simulink library "lib_drive_cycle2"  (Simulink 5.1)
values from neighbouring files (symbols this model uses):
  logFlag = 1    [advSACompMaskInit.m]    (also in advSACompMaskInitR13.m)
undefined symbols (not defined in the file or in its folder): cyc_avg_time, cyc_cargo_mass, cyc_elevation_init, cyc_filter_bool, cyc_grade, cyc_mph, veh_mass
libraries: lib_drive_cycle x2
settings Model: LastModifiedBy=mokeefe  ProdHWDeviceType=Microprocessor
settings Model: ModifiedComment=|
  | mokeefe -- Thu Apr 18 08:26:19 2002 -- Version 1.14
  | saving the model:
  | o "without the model browser open"
  | o with only top-level screen visible
  | o with "fit to view" enabled
  | o with "status bar" off and "toolbar" off
  | o with "prompt to update model history with each save" on
settings Model: ModifiedHistory=|
  | mokeefe -- Thu Apr 18 08:26:19 2002 -- Version 1.14
  | saving the model:
  | o "without the model browser open"
  | o with only top-level screen visible
  | o with "fit to view" enabled
  | o with "status bar" off and "toolbar" off
  | o with "prompt to update model history with each save" on
  | 
  | mokeefe -- Thu Apr 18 08:26:19 2002 -- Version 1.14
  | saving the model:
  | o "without the model browser open"
  | o with only top-level screen visible
  | o with "fit to view" enabled
  | o with "status bar" off and "toolbar" off
  | o with "prompt to update model history with each save" on
  | 
  | mokeefe -- Thu Apr 18 08:26:08 2002 -- Version 1.13
  | saving the model:
  | o "without the model browser open"
  | o with only top-level screen visible
  | o with "fit to view" enabled
  | o with "status bar" off and "toolbar" off
  | o with "prompt to update model history with each save" on

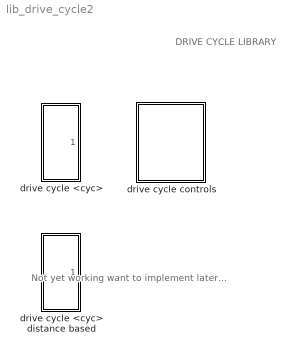
== system lib_drive_cycle2 ==
  note: DRIVE CYCLE LIBRARY
  note: Not yet working
      | want to implement
      | later...
  drive cycle <cyc> : Subsystem  mask(Stand-Alone Drive Cycle Mask){generalName='cyc', logPick=Log, initFileName={}, modCell={}, imgFileName='bdi_cyc.jpg', DEBUG=OFF, veh_mass=veh_mass}
      mask prompts: generalName "General Name of this Component [char]"; logPick "Log Variables to Workspace?"; initFileName "Initialization File(s) [cell array of char]"; modCell "Modification Cell [2 column cell array of param and val]"; imgFileName "Icon image file name [char--evaluated]"; veh_mass "Vehicle Mass (kg)"
      mask init:
      | % initialization via m-file script
      | advSACompMaskInitR13;
      mask StyleString: edit,popup(Don't Log|Log),edit,edit,edit,popup(ON|OFF),edit
      mask Display: image(imread(imgFileName))
  drive cycle <cyc> distance based : Subsystem  mask(Stand-Alone Distance-Based Drive Cycle Mask){generalName='cycd', logPick=Log, initFileName={}, modCell={}, imgFileName='bdi_cyc.jpg', DEBUG=OFF, veh_mass=veh_mass}
      mask prompts: generalName "General Name of this Component [char]"; logPick "Log Variables to Workspace?"; initFileName "Initialization File(s) [cell array of char]"; modCell "Modification Cell [2 column cell array of param and val]"; imgFileName "Icon image file name [char--evaluated]"; veh_mass "Vehicle Mass (kg)"
      mask init:
      | set_param(gcs,'StopTime','inf'); % set stop time to inf
      | % this block will stop sim when max. distance reached or max. time elapsed
      | % initialization via m-file script
      | advSACompMaskInit;
      mask StyleString: edit,popup(Don't Log|Log),edit,edit,edit,popup(ON|OFF),edit
      mask Display: image(imread(imgFileName))
  drive cycle controls : Subsystem

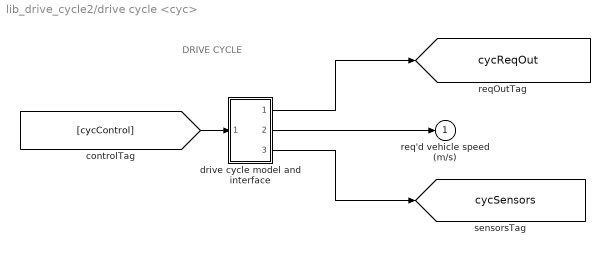
== system lib_drive_cycle2/drive cycle <cyc> ==
  note: DRIVE CYCLE
  drive cycle model and interface : Subsystem
  req'd vehicle speed (m/s) : Outport  InitialOutput=0
  tag scope: cycReqOut=global, cycSensors=global
  wires:
  drive cycle model and interface/2(req'd vehicle speed (m/s)) -> req'd vehicle speed (m/s)/1
  [cycControl] -> drive cycle model and interface/1(control)
  drive cycle model and interface/1(req'd lookups) -> [cycReqOut]
  drive cycle model and interface/3(sensors) -> [cycSensors]

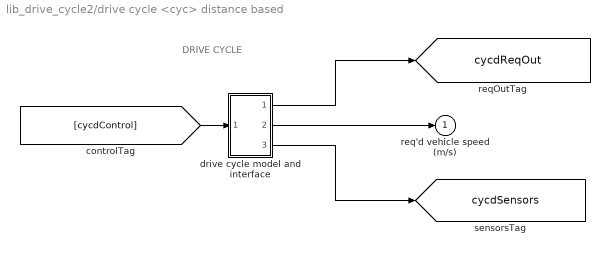
== system lib_drive_cycle2/drive cycle <cyc> distance based ==
  note: DRIVE CYCLE
  drive cycle model and interface : Subsystem
  req'd vehicle speed (m/s) : Outport  InitialOutput=0
  tag scope: cycdReqOut=global, cycdSensors=global
  wires:
  drive cycle model and interface/2(req'd vehicle speed (m/s)) -> req'd vehicle speed (m/s)/1
  [cycdControl] -> drive cycle model and interface/1(control)
  drive cycle model and interface/1(req'd vehicle speed (m/s)2) -> [cycdReqOut]
  drive cycle model and interface/3(sensors) -> [cycdSensors]

== system lib_drive_cycle2/drive cycle controls ==
  drive cycle dummy controller : Subsystem

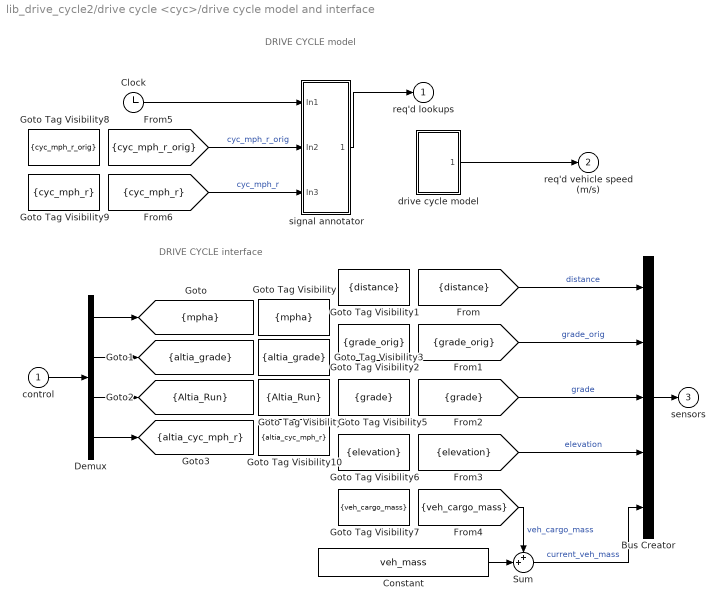
== system lib_drive_cycle2/drive cycle <cyc>/drive cycle model and interface ==
  note: DRIVE CYCLE
      | model
  note: DRIVE CYCLE
      | interface
  control : Inport
  Bus Creator : BusCreator  Inputs=5
  Clock : Clock
      settings: Decimation=10
  Constant : Constant  Value=veh_mass
  Demux : Demux
  Goto Tag Visibility : GotoTagVisibility  GotoTag=mpha
  Goto Tag Visibility1 : GotoTagVisibility  GotoTag=distance
  Goto Tag Visibility10 : GotoTagVisibility  GotoTag=altia_cyc_mph_r
  Goto Tag Visibility2 : GotoTagVisibility  GotoTag=grade_orig
  Goto Tag Visibility3 : GotoTagVisibility  GotoTag=altia_grade
  Goto Tag Visibility4 : GotoTagVisibility  GotoTag=Altia_Run
  Goto Tag Visibility5 : GotoTagVisibility  GotoTag=grade
  Goto Tag Visibility6 : GotoTagVisibility  GotoTag=elevation
  Goto Tag Visibility7 : GotoTagVisibility  GotoTag=veh_cargo_mass
  Goto Tag Visibility8 : GotoTagVisibility  GotoTag=cyc_mph_r_orig
  Goto Tag Visibility9 : GotoTagVisibility  GotoTag=cyc_mph_r
  Sum : Sum  Inputs=++|  SaturateOnIntegerOverflow=on  InputSameDT=on
  drive cycle model : Subsystem
  signal annotator : Subsystem
  req'd lookups : Outport  InitialOutput=0
  req'd vehicle speed (m/s) : Outport  Port=2  InitialOutput=0
  sensors : Outport  Port=3  InitialOutput=0
  tag scope: Altia_Run=scoped, altia_cyc_mph_r=scoped, altia_grade=scoped, mpha=scoped
  wires:
  drive cycle model/1(req'd vehicle speed (m/s)) -> req'd vehicle speed (m/s)/1
  Clock/1 -> signal annotator/1(In1)
  signal annotator/1(Out1) -> req'd lookups/1
  control/1 -> Demux/1
  Bus Creator/1 -> sensors/1
  Demux/1 -> [mpha]
  Demux/2 -> [altia_grade]
  Demux/3 -> [Altia_Run]
  Demux/4 -> [altia_cyc_mph_r]
  [distance] -> Bus Creator/1  "distance"
  [grade_orig] -> Bus Creator/2  "grade_orig"
  [grade] -> Bus Creator/3  "grade"
  [elevation] -> Bus Creator/4  "elevation"
  [veh_cargo_mass] -> Sum/1  "veh_cargo_mass"
  [cyc_mph_r_orig] -> signal annotator/2(In2)  "cyc_mph_r_orig"
  [cyc_mph_r] -> signal annotator/3(In3)  "cyc_mph_r"
  Constant/1 -> Sum/2
  Sum/1 -> Bus Creator/5  "current_veh_mass"

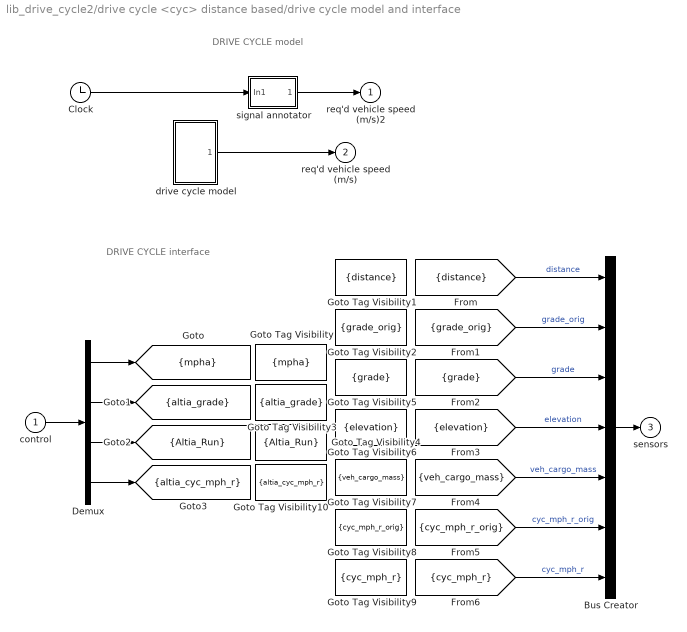
== system lib_drive_cycle2/drive cycle <cyc> distance based/drive cycle model and interface ==
  note: DRIVE CYCLE
      | model
  note: DRIVE CYCLE
      | interface
  control : Inport
  Bus Creator : BusCreator  Inputs=7
  Clock : Clock
      settings: Decimation=10
  Demux : Demux
  Goto Tag Visibility : GotoTagVisibility  GotoTag=mpha
  Goto Tag Visibility1 : GotoTagVisibility  GotoTag=distance
  Goto Tag Visibility10 : GotoTagVisibility  GotoTag=altia_cyc_mph_r
  Goto Tag Visibility2 : GotoTagVisibility  GotoTag=grade_orig
  Goto Tag Visibility3 : GotoTagVisibility  GotoTag=altia_grade
  Goto Tag Visibility4 : GotoTagVisibility  GotoTag=Altia_Run
  Goto Tag Visibility5 : GotoTagVisibility  GotoTag=grade
  Goto Tag Visibility6 : GotoTagVisibility  GotoTag=elevation
  Goto Tag Visibility7 : GotoTagVisibility  GotoTag=veh_cargo_mass
  Goto Tag Visibility8 : GotoTagVisibility  GotoTag=cyc_mph_r_orig
  Goto Tag Visibility9 : GotoTagVisibility  GotoTag=cyc_mph_r
  drive cycle model : Subsystem
  signal annotator : Subsystem
  req'd vehicle speed (m/s)2 : Outport  InitialOutput=0
  req'd vehicle speed (m/s) : Outport  Port=2  InitialOutput=0
  sensors : Outport  Port=3  InitialOutput=0
  tag scope: Altia_Run=scoped, altia_cyc_mph_r=scoped, altia_grade=scoped, mpha=scoped
  wires:
  drive cycle model/1(req'd vehicle speed (m/s)) -> req'd vehicle speed (m/s)/1
  Clock/1 -> signal annotator/1(In1)
  signal annotator/1(Out1) -> req'd vehicle speed (m/s)2/1
  control/1 -> Demux/1
  Bus Creator/1 -> sensors/1
  Demux/1 -> [mpha]
  Demux/2 -> [altia_grade]
  Demux/3 -> [Altia_Run]
  Demux/4 -> [altia_cyc_mph_r]
  [distance] -> Bus Creator/1  "distance"
  [grade_orig] -> Bus Creator/2  "grade_orig"
  [grade] -> Bus Creator/3  "grade"
  [elevation] -> Bus Creator/4  "elevation"
  [veh_cargo_mass] -> Bus Creator/5  "veh_cargo_mass"
  [cyc_mph_r_orig] -> Bus Creator/6  "cyc_mph_r_orig"
  [cyc_mph_r] -> Bus Creator/7  "cyc_mph_r"

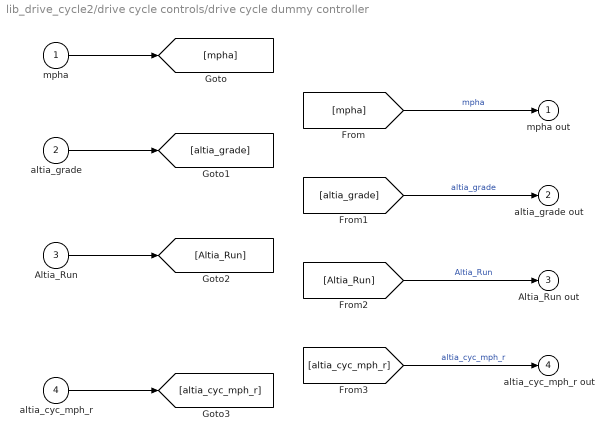
== system lib_drive_cycle2/drive cycle controls/drive cycle dummy controller ==
  mpha : Inport
  altia_grade : Inport  Port=2
  Altia_Run : Inport  Port=3
  altia_cyc_mph_r : Inport  Port=4
  mpha out : Outport  InitialOutput=0
  altia_grade out : Outport  Port=2  InitialOutput=0
  Altia_Run out : Outport  Port=3  InitialOutput=0
  altia_cyc_mph_r out : Outport  Port=4  InitialOutput=0
  wires:
  [altia_cyc_mph_r] -> altia_cyc_mph_r out/1  "altia_cyc_mph_r"
  [Altia_Run] -> Altia_Run out/1  "Altia_Run"
  [altia_grade] -> altia_grade out/1  "altia_grade"
  [mpha] -> mpha out/1  "mpha"
  altia_cyc_mph_r/1 -> [altia_cyc_mph_r]
  Altia_Run/1 -> [Altia_Run]
  altia_grade/1 -> [altia_grade]
  mpha/1 -> [mpha]

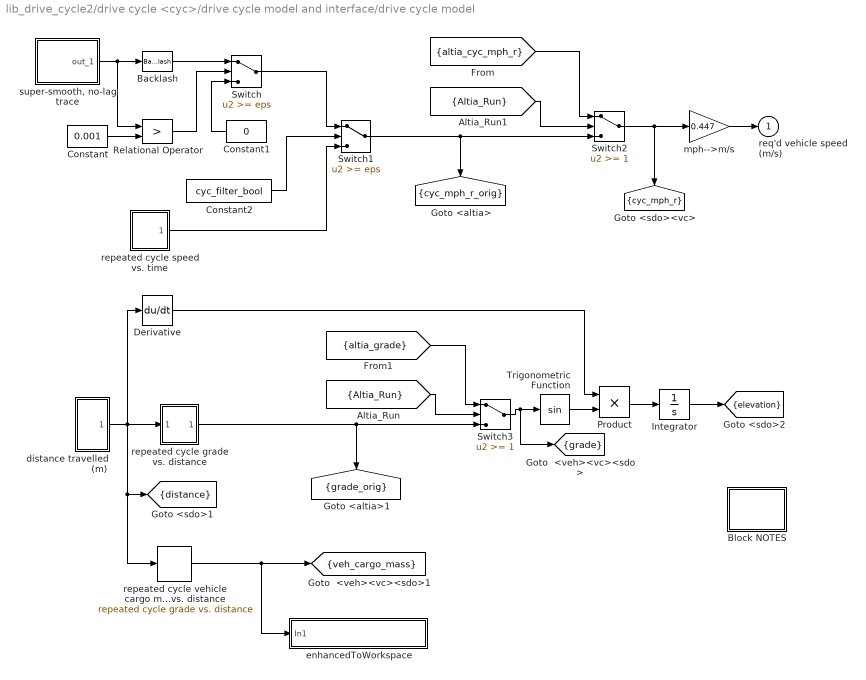
== system lib_drive_cycle2/drive cycle <cyc>/drive cycle model and interface/drive cycle model ==
  Backlash : Backlash  BacklashWidth=0.5
  Block NOTES : Subsystem
      mask Display: disp('Block\nNOTES')
  Constant : Constant  Value=0.001
  Constant1 : Constant  Orientation=left  Value=0
  Constant2 : Constant  Value=cyc_filter_bool
  Derivative : Derivative
  Integrator : Integrator  InitialCondition=cyc_elevation_init
  Product : Product  SaturateOnIntegerOverflow=on  InputSameDT=on
  Relational Operator : RelationalOperator  Operator=>  InputSameDT=on
  Switch : Switch  Threshold=eps  SaturateOnIntegerOverflow=on  InputSameDT=on
  Switch1 : Switch  Threshold=eps  SaturateOnIntegerOverflow=on  InputSameDT=on
  Switch2 : Switch  Threshold=1  SaturateOnIntegerOverflow=on  InputSameDT=on
  Switch3 : Switch  Threshold=1  SaturateOnIntegerOverflow=on  InputSameDT=on
  Trigonometric Function : Trigonometry
  distance travelled (m) : Subsystem
  enhancedToWorkspace : Subsystem  TreatAsAtomicUnit=on  mask(enhancedToWorkspace){generalName=generalName, specificName=cargo_mass_vs_time, logFlag=logFlag}
      mask prompts: generalName "General Name [char-evaluated]"; specificName "Specific Name [char-literal]"; logFlag "Enable flag (1=on,0=off)"
      mask help: A wrapper for the Simulink "To Workspace" block that allows you to evaluate the name of the variable to log to workspace. This is useful to avoid the double logging errors that occur when you pull in two library models that attempt to log to the same variable.
      mask init:
      | enhancedToWsMaker
      settings: CopyFcn=breakLinkCopyFcn  ParentCloseFcn=breakLinkParCloseFcn
      mask Help:
      | <h2>Enhanced To Workspace Block</h2>
      | <h3>Parameters</h3>
      | <UL>
      | <li><b>General Name:</b> This is the more general name of the variable. Variables are saved to the workspace as <i>generalName_specificName</i>. Note that this is an evaluated variable. If you would like to type in the value directly, it must be surrounded with single quotes. Otherwise you can input the name of a variable containing a char string.</li>
      | <li><b>Specific Name:</b> This is the specific name of the variable. Note that this is input as a char literal (i.e., you don't need quotes).</li>
      | <li><b>Enable Flag:</b> This flag should have the value of 0 or 1. If 0, the variable will not be logged to the workspace. If 1, the variable will be logged. This is done so that variable logging can be turned off to improve speed.</li>
      | </ul>
      | <h3>Overview</h3>
      | <p>The enhanced to workspace block was put together to allow one to dynamically resolve variable names at run time in simulink. This is most powerful when used in conjunction with a masked subsystem to allow multiple instances of that masked subsytem to be used in the same model. The strategy is to set the generalName in the block mask which will allow the block to change the general name for all variable logging on the fly.
      | <h3>Helper Files</h3>
      | <p>Three m-files are required by the enhancedToWorkspace block. These files are located in the &lt; ADVISOR root &gt;/GUI directory :
      | <ul>
      | <li><i>enhancedToWsMaker.m</i> This file runs the mask initialization for the block</li>
      | <li><i>breakLinkCopyFcn.m</i> This file is used by the block callback when the simulink block is copied. It is necessary to break the link to the enhancedToWorkspace similar to the To Workspace block in order for it to be able to configure itself. (Try copying simulink's To Workspace block--it is impossible to make a link)</li>
      | <li><i>breakLinkParCloseFcn.m</i> This file is similar to the breakLinkCopyFcn and is used when a parent system is closed</li>
      | </ul>
      | <hr>
      | 
      | <p>Created 2003-Jan-21, Michael Patrick O'Keefe, NREL</p>
      | 
      | <!--
      | <VARDEF>
      | <H3>var_name</H3>
      | <UL>
      | <LI><B>data type</B> data type here</LI>
      | <LI><B>units</B> units here</LI>
      | <LI><B>vehicle type</B> vehicle type here</LI>
      | <LI><B>description</B> description here</LI>
      | </UL>
      | </VARDEF>
      | -->
      mask Display: disp([generalName,'_',specificName])
  mph-->m/s : Gain  Gain=0.447  SaturateOnIntegerOverflow=on
  repeated cycle grade vs. distance : Subsystem  mask(Repeating table){t=cyc_grade(:,1), y=cyc_grade(:,2)}
      mask prompts: t "Input values:"; y "Output values:"
      mask help:
      | Repeating table.
      | Enter values of input and output for first cycle.
      mask init:
      | period = max(@1);
      mask Help: Repeats cycle given in table. Input values should be monotonically increasing.
  repeated cycle speed vs. time : Subsystem  mask(Repeating table){@1=cyc_mph(:,1), @2=cyc_mph(:,2)}
      mask prompts: @1 "Time values:"; @2 "Output values:"
      mask help:
      | Repeating table.
      | Enter values of time and output for first cycle.
      mask init:
      | period = max(@1); t = @1; y = @2;
      mask Help: Repeats cycle given in table. Time values should be monotonically increasing.
  repeated cycle vehicle cargo mass vs. distance : lib_drive_cycle/drive cycle <cyc>/repeated cycle grade vs. distance  t=cyc_cargo_mass(:,1)  y=cyc_cargo_mass(:,2)
  "super-smooth, no-lag trace" : Subsystem  mask(Smooth Cycle){t=cyc_mph(:,1), y=cyc_mph(:,2), avgtime=cyc_avg_time}
      mask prompts: t "Time vector for trace (s):"; y "Speed vector for trace (km/hr):"; avgtime "Averaging time (s):"
      mask help: Smooth Cycle
      mask init:
      | period = max(@1);,
      mask Display: disp('SMOOTH\nCYCLE')
  req'd vehicle speed (m/s) : Outport  InitialOutput=0
  tag scope: cyc_mph_r=scoped, cyc_mph_r_orig=scoped, distance=scoped, elevation=scoped, grade=scoped, grade_orig=scoped, veh_cargo_mass=scoped
  wires:
  repeated cycle grade vs. distance/1(out_1) -> [grade_orig], Switch3/3
  distance travelled (m)/1(Out1) -> repeated cycle grade vs. distance/1(distance travelled (m)), Derivative/1, [distance], repeated cycle vehicle cargo mass vs. distance/1
  Switch3/1 -> Trigonometric Function/1, [grade]
  Integrator/1 -> [elevation]
  Trigonometric Function/1 -> Product/2
  Derivative/1 -> Product/1
  Product/1 -> Integrator/1
  Switch1/1 -> Switch2/3, [cyc_mph_r_orig]
  repeated cycle speed vs. time/1(out_1) -> Switch1/3
  Switch/1 -> Switch1/1
  "super-smooth, no-lag trace"/1(out_1) -> Backlash/1, Relational Operator/1
  Constant/1 -> Relational Operator/2
  Backlash/1 -> Switch/1
  Relational Operator/1 -> Switch/2
  Constant1/1 -> Switch/3
  Constant2/1 -> Switch1/2
  Switch2/1 -> [cyc_mph_r], mph-->m/s/1
  mph-->m/s/1 -> req'd vehicle speed (m/s)/1
  [altia_cyc_mph_r] -> Switch2/1
  [Altia_Run] -> Switch2/2
  [altia_grade] -> Switch3/1
  [Altia_Run] -> Switch3/2
  repeated cycle vehicle cargo mass vs. distance/1 -> [veh_cargo_mass], enhancedToWorkspace/1(In1)

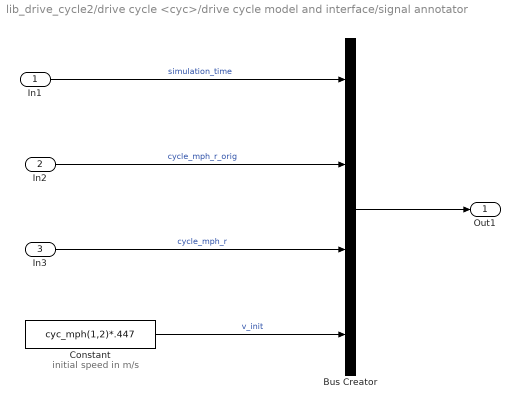
== system lib_drive_cycle2/drive cycle <cyc>/drive cycle model and interface/signal annotator ==
  note: initial speed in m/s
  In1 : Inport
  In2 : Inport  Port=2
  In3 : Inport  Port=3
  Bus Creator : BusCreator
  Constant : Constant  Value=cyc_mph(1,2)*.447
  Out1 : Outport
  wires:
  In1/1 -> Bus Creator/1  "simulation_time"
  Bus Creator/1 -> Out1/1
  In2/1 -> Bus Creator/2  "cycle_mph_r_orig"
  In3/1 -> Bus Creator/3  "cycle_mph_r"
  Constant/1 -> Bus Creator/4  "v_init"

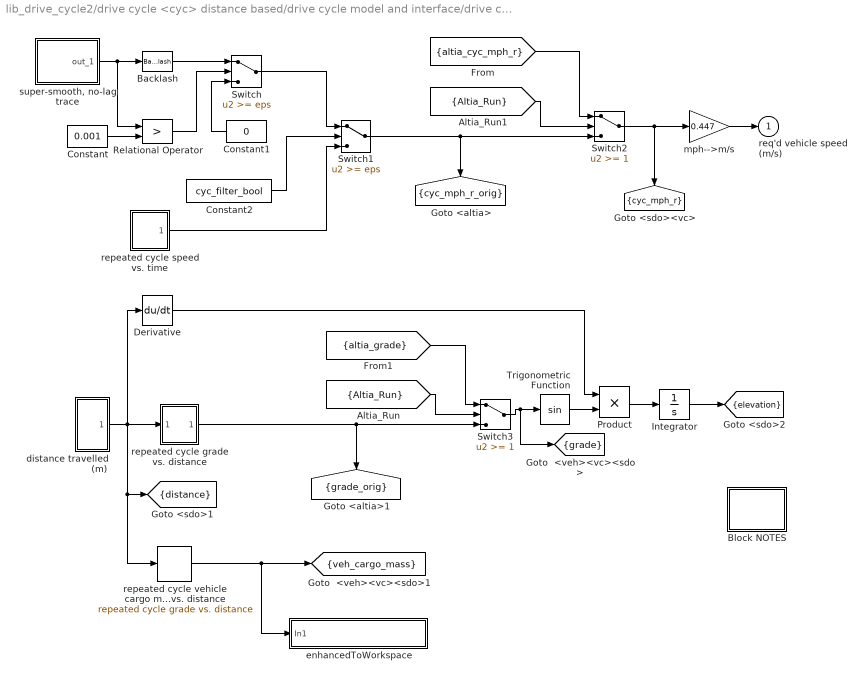
== system lib_drive_cycle2/drive cycle <cyc> distance based/drive cycle model and interface/drive cycle model ==
  Backlash : Backlash  BacklashWidth=0.5
  Block NOTES : Subsystem
      mask Display: disp('Block\nNOTES')
  Constant : Constant  Value=0.001
  Constant1 : Constant  Orientation=left  Value=0
  Constant2 : Constant  Value=cyc_filter_bool
  Derivative : Derivative
  Integrator : Integrator  InitialCondition=cyc_elevation_init
  Product : Product  SaturateOnIntegerOverflow=on  InputSameDT=on
  Relational Operator : RelationalOperator  Operator=>  InputSameDT=on
  Switch : Switch  Threshold=eps  SaturateOnIntegerOverflow=on  InputSameDT=on
  Switch1 : Switch  Threshold=eps  SaturateOnIntegerOverflow=on  InputSameDT=on
  Switch2 : Switch  Threshold=1  SaturateOnIntegerOverflow=on  InputSameDT=on
  Switch3 : Switch  Threshold=1  SaturateOnIntegerOverflow=on  InputSameDT=on
  Trigonometric Function : Trigonometry
  distance travelled (m) : Subsystem
  enhancedToWorkspace : Subsystem  TreatAsAtomicUnit=on  mask(enhancedToWorkspace){generalName=generalName, specificName=cargo_mass_vs_time, logFlag=logFlag}
      mask prompts: generalName "General Name [char-evaluated]"; specificName "Specific Name [char-literal]"; logFlag "Enable flag (1=on,0=off)"
      mask help: A wrapper for the Simulink "To Workspace" block that allows you to evaluate the name of the variable to log to workspace. This is useful to avoid the double logging errors that occur when you pull in two library models that attempt to log to the same variable.
      mask init:
      | enhancedToWsMaker
      settings: CopyFcn=breakLinkCopyFcn  ParentCloseFcn=breakLinkParCloseFcn
      mask Help:
      | <h2>Enhanced To Workspace Block</h2>
      | <h3>Parameters</h3>
      | <UL>
      | <li><b>General Name:</b> This is the more general name of the variable. Variables are saved to the workspace as <i>generalName_specificName</i>. Note that this is an evaluated variable. If you would like to type in the value directly, it must be surrounded with single quotes. Otherwise you can input the name of a variable containing a char string.</li>
      | <li><b>Specific Name:</b> This is the specific name of the variable. Note that this is input as a char literal (i.e., you don't need quotes).</li>
      | <li><b>Enable Flag:</b> This flag should have the value of 0 or 1. If 0, the variable will not be logged to the workspace. If 1, the variable will be logged. This is done so that variable logging can be turned off to improve speed.</li>
      | </ul>
      | <h3>Overview</h3>
      | <p>The enhanced to workspace block was put together to allow one to dynamically resolve variable names at run time in simulink. This is most powerful when used in conjunction with a masked subsystem to allow multiple instances of that masked subsytem to be used in the same model. The strategy is to set the generalName in the block mask which will allow the block to change the general name for all variable logging on the fly.
      | <h3>Helper Files</h3>
      | <p>Three m-files are required by the enhancedToWorkspace block. These files are located in the &lt; ADVISOR root &gt;/GUI directory :
      | <ul>
      | <li><i>enhancedToWsMaker.m</i> This file runs the mask initialization for the block</li>
      | <li><i>breakLinkCopyFcn.m</i> This file is used by the block callback when the simulink block is copied. It is necessary to break the link to the enhancedToWorkspace similar to the To Workspace block in order for it to be able to configure itself. (Try copying simulink's To Workspace block--it is impossible to make a link)</li>
      | <li><i>breakLinkParCloseFcn.m</i> This file is similar to the breakLinkCopyFcn and is used when a parent system is closed</li>
      | </ul>
      | <hr>
      | 
      | <p>Created 2003-Jan-21, Michael Patrick O'Keefe, NREL</p>
      | 
      | <!--
      | <VARDEF>
      | <H3>var_name</H3>
      | <UL>
      | <LI><B>data type</B> data type here</LI>
      | <LI><B>units</B> units here</LI>
      | <LI><B>vehicle type</B> vehicle type here</LI>
      | <LI><B>description</B> description here</LI>
      | </UL>
      | </VARDEF>
      | -->
      mask Display: disp([generalName,'_',specificName])
  mph-->m/s : Gain  Gain=0.447  SaturateOnIntegerOverflow=on
  repeated cycle grade vs. distance : Subsystem  mask(Repeating table){t=cyc_grade(:,1), y=cyc_grade(:,2)}
      mask prompts: t "Input values:"; y "Output values:"
      mask help:
      | Repeating table.
      | Enter values of input and output for first cycle.
      mask init:
      | period = max(@1);
      mask Help: Repeats cycle given in table. Input values should be monotonically increasing.
  repeated cycle speed vs. time : Subsystem  mask(Repeating table){@1=cyc_mph(:,1), @2=cyc_mph(:,2)}
      mask prompts: @1 "Time values:"; @2 "Output values:"
      mask help:
      | Repeating table.
      | Enter values of time and output for first cycle.
      mask init:
      | period = max(@1); t = @1; y = @2;
      mask Help: Repeats cycle given in table. Time values should be monotonically increasing.
  repeated cycle vehicle cargo mass vs. distance : lib_drive_cycle/drive cycle <cyc>/repeated cycle grade vs. distance  t=cyc_cargo_mass(:,1)  y=cyc_cargo_mass(:,2)
  "super-smooth, no-lag trace" : Subsystem  mask(Smooth Cycle){t=cyc_mph(:,1), y=cyc_mph(:,2), avgtime=cyc_avg_time}
      mask prompts: t "Time vector for trace (s):"; y "Speed vector for trace (km/hr):"; avgtime "Averaging time (s):"
      mask help: Smooth Cycle
      mask init:
      | period = max(@1);,
      mask Display: disp('SMOOTH\nCYCLE')
  req'd vehicle speed (m/s) : Outport  InitialOutput=0
  tag scope: cyc_mph_r=scoped, cyc_mph_r_orig=scoped, distance=scoped, elevation=scoped, grade=scoped, grade_orig=scoped, veh_cargo_mass=scoped
  wires:
  repeated cycle grade vs. distance/1(out_1) -> [grade_orig], Switch3/3
  distance travelled (m)/1(Out1) -> repeated cycle grade vs. distance/1(distance travelled (m)), Derivative/1, [distance], repeated cycle vehicle cargo mass vs. distance/1
  Switch3/1 -> Trigonometric Function/1, [grade]
  Integrator/1 -> [elevation]
  Trigonometric Function/1 -> Product/2
  Derivative/1 -> Product/1
  Product/1 -> Integrator/1
  Switch1/1 -> Switch2/3, [cyc_mph_r_orig]
  repeated cycle speed vs. time/1(out_1) -> Switch1/3
  Switch/1 -> Switch1/1
  "super-smooth, no-lag trace"/1(out_1) -> Backlash/1, Relational Operator/1
  Constant/1 -> Relational Operator/2
  Backlash/1 -> Switch/1
  Relational Operator/1 -> Switch/2
  Constant1/1 -> Switch/3
  Constant2/1 -> Switch1/2
  Switch2/1 -> [cyc_mph_r], mph-->m/s/1
  mph-->m/s/1 -> req'd vehicle speed (m/s)/1
  [altia_cyc_mph_r] -> Switch2/1
  [Altia_Run] -> Switch2/2
  [altia_grade] -> Switch3/1
  [Altia_Run] -> Switch3/2
  repeated cycle vehicle cargo mass vs. distance/1 -> [veh_cargo_mass], enhancedToWorkspace/1(In1)

== system lib_drive_cycle2/drive cycle <cyc> distance based/drive cycle model and interface/signal annotator ==
  In1 : Inport
  Out1 : Outport
  wires:
  In1/1 -> Out1/1  "simulation_time"

== system lib_drive_cycle2/drive cycle <cyc>/drive cycle model and interface/drive cycle model/Block NOTES ==
  note: This block determines the speed required of the vehicle.  If cyc_filter_bool
      | is true, a centered-in-time average of the trace, with backlash, is required of
      | the vehicle.  This may be useful to smooth out jumps in the trace.  Otherwise,
      | the trace, exactly as published, is required of the vehicle.
      | This block also determines the roadway grade of the cycle and the
      | elevation as a function of the distance travelelled

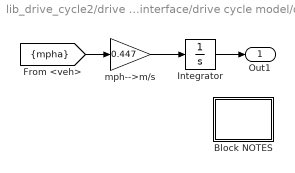
== system lib_drive_cycle2/drive cycle <cyc>/drive cycle model and interface/drive cycle model/distance travelled (m) ==
  Block NOTES : Subsystem
      mask Display: disp('Block\nNOTES')
  Integrator : Integrator
  mph-->m/s : Gain  Gain=0.447  SaturateOnIntegerOverflow=on
  Out1 : Outport  InitialOutput=0
  wires:
  Integrator/1 -> Out1/1
  [mpha] -> mph-->m/s/1
  mph-->m/s/1 -> Integrator/1

== system lib_drive_cycle2/drive cycle <cyc>/drive cycle model and interface/drive cycle model/enhancedToWorkspace ==
  In1 : Inport
  To Workspace : ToWorkspace  VariableName=cyc_cargo_mass_vs_time  SampleTime=-1  SaveFormat=Array
  wires:
  In1/1 -> To Workspace/1

== system lib_drive_cycle2/drive cycle <cyc>/drive cycle model and interface/drive cycle model/repeated cycle grade vs. distance ==
  distance travelled (m) : Inport
  Fcn1 : Fcn  Expr=rem(u[1],period)
  Look-Up Table : Lookup  InputValues=t  OutputValues=y  SaturateOnIntegerOverflow=on
  out_1 : Outport  InitialOutput=0
  wires:
  distance travelled (m)/1 -> Fcn1/1
  Fcn1/1 -> Look-Up Table/1
  Look-Up Table/1 -> out_1/1

== system lib_drive_cycle2/drive cycle <cyc>/drive cycle model and interface/drive cycle model/repeated cycle speed vs. time ==
  Clock : Clock
      settings: Decimation=10
  Fcn1 : Fcn  Expr=rem(u[1],period)
  Look-Up Table : Lookup  InputValues=t  OutputValues=y  SaturateOnIntegerOverflow=on
  out_1 : Outport  InitialOutput=0
  wires:
  Fcn1/1 -> Look-Up Table/1
  Clock/1 -> Fcn1/1
  Look-Up Table/1 -> out_1/1

== system lib_drive_cycle2/drive cycle <cyc>/drive cycle model and interface/drive cycle model/super-smooth, no-lag trace ==
  Subsystem : Subsystem  mask(Running Average){@1=avgtime}
      mask prompts: @1 "Averaging Time (s)"
      mask help: Running Average
      mask init:
      | n=@1;
      mask Help: Output is the average of the last (Averaging Time) seconds of input.
      mask Display: disp('Running\nAverage')
  repeated cycle : Subsystem
  out_1 : Outport  InitialOutput=0
  wires:
  Subsystem/1(out_1) -> out_1/1
  repeated cycle/1(out_1) -> Subsystem/1(in_1)

== system lib_drive_cycle2/drive cycle <cyc> distance based/drive cycle model and interface/drive cycle model/Block NOTES ==
  note: This block determines the speed required of the vehicle.  If cyc_filter_bool
      | is true, a centered-in-time average of the trace, with backlash, is required of
      | the vehicle.  This may be useful to smooth out jumps in the trace.  Otherwise,
      | the trace, exactly as published, is required of the vehicle.
      | This block also determines the roadway grade of the cycle and the
      | elevation as a function of the distance travelelled

== system lib_drive_cycle2/drive cycle <cyc> distance based/drive cycle model and interface/drive cycle model/distance travelled (m) ==
  Block NOTES : Subsystem
      mask Display: disp('Block\nNOTES')
  Integrator : Integrator
  mph-->m/s : Gain  Gain=0.447  SaturateOnIntegerOverflow=on
  Out1 : Outport  InitialOutput=0
  wires:
  Integrator/1 -> Out1/1
  [mpha] -> mph-->m/s/1
  mph-->m/s/1 -> Integrator/1

== system lib_drive_cycle2/drive cycle <cyc> distance based/drive cycle model and interface/drive cycle model/enhancedToWorkspace ==
  In1 : Inport
  To Workspace : ToWorkspace  VariableName=cyc_cargo_mass_vs_time  SampleTime=-1  SaveFormat=Array
  wires:
  In1/1 -> To Workspace/1

== system lib_drive_cycle2/drive cycle <cyc> distance based/drive cycle model and interface/drive cycle model/repeated cycle grade vs. distance ==
  distance travelled (m) : Inport
  Fcn1 : Fcn  Expr=rem(u[1],period)
  Look-Up Table : Lookup  InputValues=t  OutputValues=y  SaturateOnIntegerOverflow=on
  out_1 : Outport  InitialOutput=0
  wires:
  distance travelled (m)/1 -> Fcn1/1
  Fcn1/1 -> Look-Up Table/1
  Look-Up Table/1 -> out_1/1

== system lib_drive_cycle2/drive cycle <cyc> distance based/drive cycle model and interface/drive cycle model/repeated cycle speed vs. time ==
  Clock : Clock
      settings: Decimation=10
  Fcn1 : Fcn  Expr=rem(u[1],period)
  Look-Up Table : Lookup  InputValues=t  OutputValues=y  SaturateOnIntegerOverflow=on
  out_1 : Outport  InitialOutput=0
  wires:
  Fcn1/1 -> Look-Up Table/1
  Clock/1 -> Fcn1/1
  Look-Up Table/1 -> out_1/1

== system lib_drive_cycle2/drive cycle <cyc> distance based/drive cycle model and interface/drive cycle model/super-smooth, no-lag trace ==
  Subsystem : Subsystem  mask(Running Average){@1=avgtime}
      mask prompts: @1 "Averaging Time (s)"
      mask help: Running Average
      mask init:
      | n=@1;
      mask Help: Output is the average of the last (Averaging Time) seconds of input.
      mask Display: disp('Running\nAverage')
  repeated cycle : Subsystem
  out_1 : Outport  InitialOutput=0
  wires:
  Subsystem/1(out_1) -> out_1/1
  repeated cycle/1(out_1) -> Subsystem/1(in_1)

== system lib_drive_cycle2/drive cycle <cyc>/drive cycle model and interface/drive cycle model/distance travelled (m)/Block NOTES ==
  note: This block calculates the distance travelled by the
      |  vehicle based on the achieved speed.

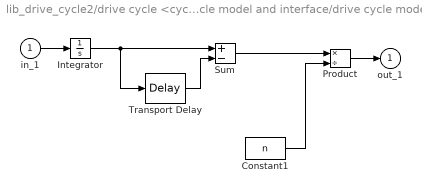
== system lib_drive_cycle2/drive cycle <cyc>/drive cycle model and interface/drive cycle model/super-smooth, no-lag trace/Subsystem ==
  in_1 : Inport
  Constant1 : Constant  Value=n
  Integrator : Integrator
  Product : Product  Inputs=*/  SaturateOnIntegerOverflow=on  InputSameDT=on
  Sum : Sum  Inputs=+-  SaturateOnIntegerOverflow=on  InputSameDT=on
  Transport Delay : TransportDelay  DelayTime=n
  out_1 : Outport  InitialOutput=0
  wires:
  Constant1/1 -> Product/2
  Product/1 -> out_1/1
  in_1/1 -> Integrator/1
  Sum/1 -> Product/1
  Transport Delay/1 -> Sum/2
  Integrator/1 -> Transport Delay/1, Sum/1

== system lib_drive_cycle2/drive cycle <cyc>/drive cycle model and interface/drive cycle model/super-smooth, no-lag trace/repeated cycle ==
  Clock : Clock
      settings: Decimation=10
  Fcn1 : Fcn  Expr=rem(u+avgtime*0.75,period)
  Look-Up Table : Lookup  InputValues=t  OutputValues=y  SaturateOnIntegerOverflow=on
  out_1 : Outport  InitialOutput=0
  wires:
  Look-Up Table/1 -> out_1/1
  Clock/1 -> Fcn1/1
  Fcn1/1 -> Look-Up Table/1

== system lib_drive_cycle2/drive cycle <cyc> distance based/drive cycle model and interface/drive cycle model/distance travelled (m)/Block NOTES ==
  note: This block calculates the distance travelled by the
      |  vehicle based on the achieved speed.

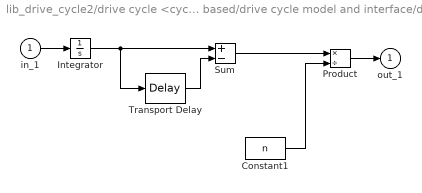
== system lib_drive_cycle2/drive cycle <cyc> distance based/drive cycle model and interface/drive cycle model/super-smooth, no-lag trace/Subsystem ==
  in_1 : Inport
  Constant1 : Constant  Value=n
  Integrator : Integrator
  Product : Product  Inputs=*/  SaturateOnIntegerOverflow=on  InputSameDT=on
  Sum : Sum  Inputs=+-  SaturateOnIntegerOverflow=on  InputSameDT=on
  Transport Delay : TransportDelay  DelayTime=n
  out_1 : Outport  InitialOutput=0
  wires:
  Constant1/1 -> Product/2
  Product/1 -> out_1/1
  in_1/1 -> Integrator/1
  Sum/1 -> Product/1
  Transport Delay/1 -> Sum/2
  Integrator/1 -> Transport Delay/1, Sum/1

== system lib_drive_cycle2/drive cycle <cyc> distance based/drive cycle model and interface/drive cycle model/super-smooth, no-lag trace/repeated cycle ==
  Clock : Clock
      settings: Decimation=10
  Fcn1 : Fcn  Expr=rem(u+avgtime*0.75,period)
  Look-Up Table : Lookup  InputValues=t  OutputValues=y  SaturateOnIntegerOverflow=on
  out_1 : Outport  InitialOutput=0
  wires:
  Look-Up Table/1 -> out_1/1
  Clock/1 -> Fcn1/1
  Fcn1/1 -> Look-Up Table/1
